simulink model "TWOLEVELFINAL"  (Simulink 7.3)
settings: Solver=ode3  StartTime=0.0  StopTime=0.5  FixedStep=1e-5  RelTol=1e-3
libraries: powerlib x14, simulink x1
settings Model: Creator=SAI GOWTHAM TEJA  LastModifiedBy=SAI GOWTHAM TEJA

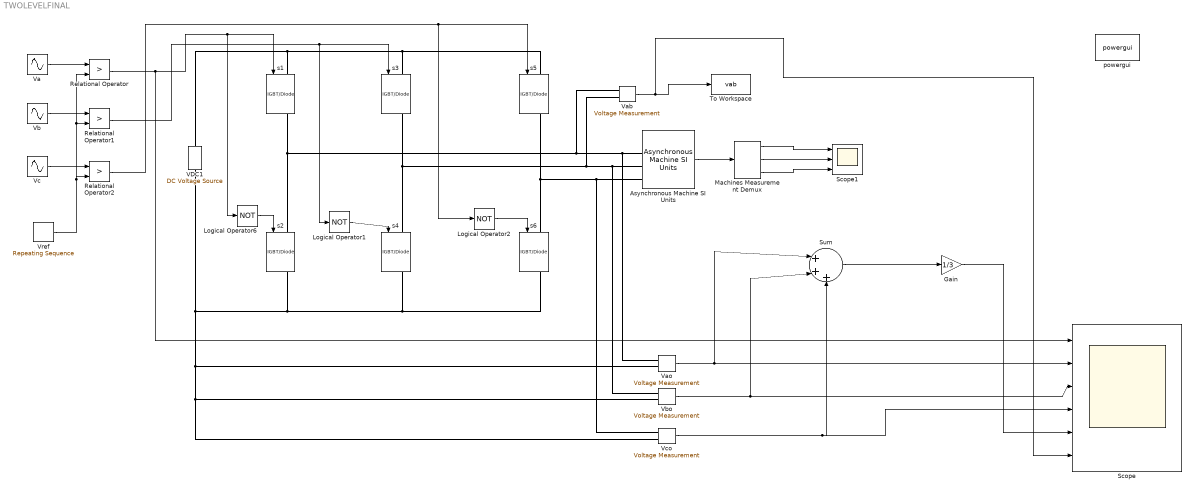
== system TWOLEVELFINAL ==
  Asynchronous Machine SI Units : powerlib/Machines/Asynchronous Machine SI Units  DialogController=POWERSYS.PowerSysDialog  SystemSampleTime=-1  PresetModel="15:  5.4 HP (4KW)   400 V  50Hz 1430 RPM"  MechanicalLoad=Torque Tm  ShowDetailedParameters=on  RotorType=Squirrel-cage  ReferenceFrame=Stationary  NominalParameters=[4000 400 50]  Stator=[1.405 0.005839]  Rotor=[1.395 0.005839]  Lm=0.1722  Mechanical=[0.0131 0.002985 2]  PolePairs=2  InitialConditions=[1 0 0 0 0 0 0 0]  Units=SI  LoadFlowParameters=1492000  SimulateSaturation=off  Saturation=[14.03593122, 27.81365428, 53.79336849, 72.68890987, 97.98006896, 148.6815601, 215.7428561, 302.9841135, 428.7778367 ; 230, 322, 414, 460, 506, 552, 598, 644, 690]  TsPowergui=0  TsBlock=-1  IterativeModel=Forward Euler
  Gain : Gain  Gain=1/3  ParameterDataType=fixdt(1, 16)  ParameterScaling=2^0  OutDataType=fixdt(1, 16)  OutScaling=2^0
  Logical Operator1 : Logic  Operator=NOT  AllPortsSameDT=off  OutDataTypeMode=boolean  LogicDataType=fixdt(0, 8)  OutDataTypeStr=boolean
  Logical Operator2 : Logic  Operator=NOT  AllPortsSameDT=off  OutDataTypeMode=boolean  LogicDataType=fixdt(0, 8)  OutDataTypeStr=boolean
  Logical Operator6 : Logic  Operator=NOT  AllPortsSameDT=off  OutDataTypeMode=boolean  LogicDataType=fixdt(0, 8)  OutDataTypeStr=boolean
  Machines Measurement Demux : powerlib/Machines/Machines Measurement Demux  DialogController=POWERSYS.PowerSysDialog  SystemSampleTime=-1  machType=Asynchronous  ssm1=on  ssm2=on  ssm3=on  ssm4=on  ssm5=on  ssm6=on  sm1=off  sm2=off  sm3=off  sm4=off  sm5=off  sm6=off  sm7=off  sm8=on  sm9=off  sm10=off  sm11=off  sm115=off  sm12=off  sm13=off  sm14=off  asm1=off  asm2=off  asm3=off  asm4=off  asm5=on  asm6=off  asm7=off  asm8=off  asm9=on  asm10=on  asm11=off  pmsm1=on  pmsm2=on  pmsm3=on  pmsm4=off  pmsm5=on  pmsm6=on  pmsm7=on  lastType=1
  Relational Operator : RelationalOperator  Operator=>  LogicOutDataTypeMode=boolean  LogicDataType=fixdt(0, 8)  OutDataTypeStr=boolean
  Relational Operator1 : RelationalOperator  Operator=>  LogicOutDataTypeMode=boolean  LogicDataType=fixdt(0, 8)  OutDataTypeStr=boolean
  Relational Operator2 : RelationalOperator  Operator=>  LogicOutDataTypeMode=boolean  LogicDataType=fixdt(0, 8)  OutDataTypeStr=boolean
  Scope : Scope  NumInputPorts=6
      settings: YMin=-5~-5~-5~-5~-5~-5  YMax=5~5~5~5~5~5
  Scope1 : Scope  NumInputPorts=3
      settings: YMin=-5~-5~-5  YMax=5~5~5
  Sum : Sum  Inputs=|+++  OutDataType=fixdt(1, 16)  OutScaling=2^0
  To Workspace : ToWorkspace  VariableName=vab  SampleTime=-1  SaveFormat=Structure With Time
  VDC1 : powerlib/Electrical Sources/DC Voltage Source  DialogController=POWERSYS.PowerSysDialog  SystemSampleTime=-1  Amplitude=510  Measurements=None
  Va : Sin  Amplitude=0.9  Bias=0  Frequency=2*pi*50  Phase=0  Samples=10  SampleTime=0  Offset=0
  Vab : powerlib/Measurements/Voltage Measurement  DialogController=POWERSYS.PowerSysDialog  SystemSampleTime=-1  PhasorSimulation=off  OutputType=Complex  PSBequivalent=0
  Vao : powerlib/Measurements/Voltage Measurement  DialogController=POWERSYS.PowerSysDialog  SystemSampleTime=-1  PhasorSimulation=off  OutputType=Complex  PSBequivalent=0
  Vb : Sin  Amplitude=0.9  Bias=0  Frequency=2*pi*50  Phase=-2*pi/3  Samples=10  SampleTime=0  Offset=0
  Vbo : powerlib/Measurements/Voltage Measurement  DialogController=POWERSYS.PowerSysDialog  SystemSampleTime=-1  PhasorSimulation=off  OutputType=Complex  PSBequivalent=0
  Vc : Sin  Amplitude=0.9  Bias=0  Frequency=2*pi*50  Phase=-4*pi/3  Samples=10  SampleTime=0  Offset=0
  Vco : powerlib/Measurements/Voltage Measurement  DialogController=POWERSYS.PowerSysDialog  SystemSampleTime=-1  PhasorSimulation=off  OutputType=Complex  PSBequivalent=0
  Vref : simulink/Sources/Repeating Sequence  SystemSampleTime=-1  rep_seq_t=[0 0.5/3000 1/3000]  rep_seq_y="[-1  1 -1]"
  powergui : powerlib/powergui  Priority=1  SystemSampleTime=-1  SimulationMode=Continuous  SampleTime=50e-6  frequency=60  SPID=off  DisableSnubberDevices=off  DisableRonSwitches=off  DisableVfSwitches=off  SwTol=0  Interpol=off  frequencyindice=0  echomessages=off  HookPort=off  DisplayEquations=off  FunctionMessages=off  EnableUseOfTLC=off  x0status=blocks  RestoreLinks=warning  Frange=[0:2:500]  Ylog=off  Xlog=on  ShowGrid=off  save=off  variable=ZData  structure=vab  ZoomFFT=off  StartTime=0.3  cycles=1  DisplayStyle=1  fundamental=50  FreqAxis=off  MaxFrequency=9000  frequencyindicesteady=1  RmsSteady=1  display=off  Ts=0  methode=off
  s{1..6} (6 alike) : powerlib/Power Electronics/IGBT//Diode  DialogController=POWERSYS.PowerSysDialog  SystemSampleTime=-1  Ron=1e-3  Rs=1e5  Cs=inf  Measurements=on
  wires:
  Va/1 -> Relational Operator/1
  Vb/1 -> Relational Operator1/1
  Vc/1 -> Relational Operator2/1
  Vref/1 -> Relational Operator/2, Relational Operator1/2, Relational Operator2/2
  Relational Operator/1 -> s1/1, Logical Operator6/1, Scope/1
  Relational Operator1/1 -> s3/1, Logical Operator1/1
  Relational Operator2/1 -> s5/1, Logical Operator2/1
  Logical Operator1/1 -> s4/1
  Logical Operator2/1 -> s6/1
  Logical Operator6/1 -> s2/1
  Vao/1 -> Sum/1, Scope/2
  Asynchronous Machine SI Units/1 -> Machines Measurement Demux/1
  Machines Measurement Demux/1 -> Scope1/1
  Machines Measurement Demux/2 -> Scope1/2
  Machines Measurement Demux/3 -> Scope1/3
  Vbo/1 -> Sum/2, Scope/3
  Vco/1 -> Sum/3, Scope/4
  Sum/1 -> Gain/1
  Vab/1 -> To Workspace/1, Scope/6
  Gain/1 -> Scope/5
  connections:
  s1/LConn1 -- s3/LConn1 -- s5/LConn1 -- VDC1/RConn1
  s6/LConn1 -- s5/RConn1 -- Asynchronous Machine SI Units/LConn3 -- Vco/LConn1
  s4/LConn1 -- s3/RConn1 -- Asynchronous Machine SI Units/LConn2 -- Vbo/LConn1 -- Vab/LConn2
  s1/RConn1 -- s2/LConn1 -- Asynchronous Machine SI Units/LConn1 -- Vao/LConn1 -- Vab/LConn1
  s6/RConn1 -- s4/RConn1 -- s2/RConn1 -- VDC1/LConn1 -- Vao/LConn2 -- Vbo/LConn2 -- Vco/LConn2
